simulink model "m060_HeaterAndBucket"  (R2022a)
settings: Solver=VariableStepAuto  StartTime=0.0  StopTime=500  RelTol=1e-3
settings Model: Creator=Admin  LastModifiedBy=Admin

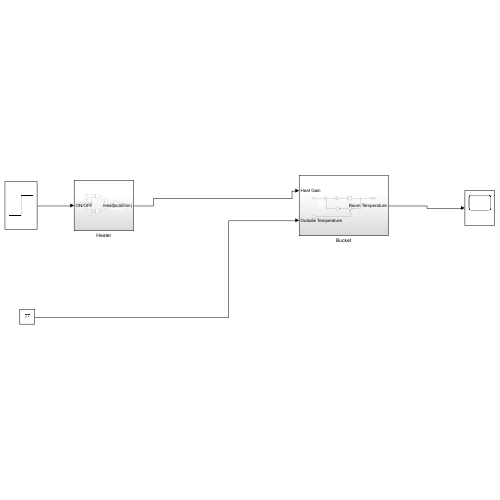
[thumbnail: Simulink's stored preview of the top-level diagram]
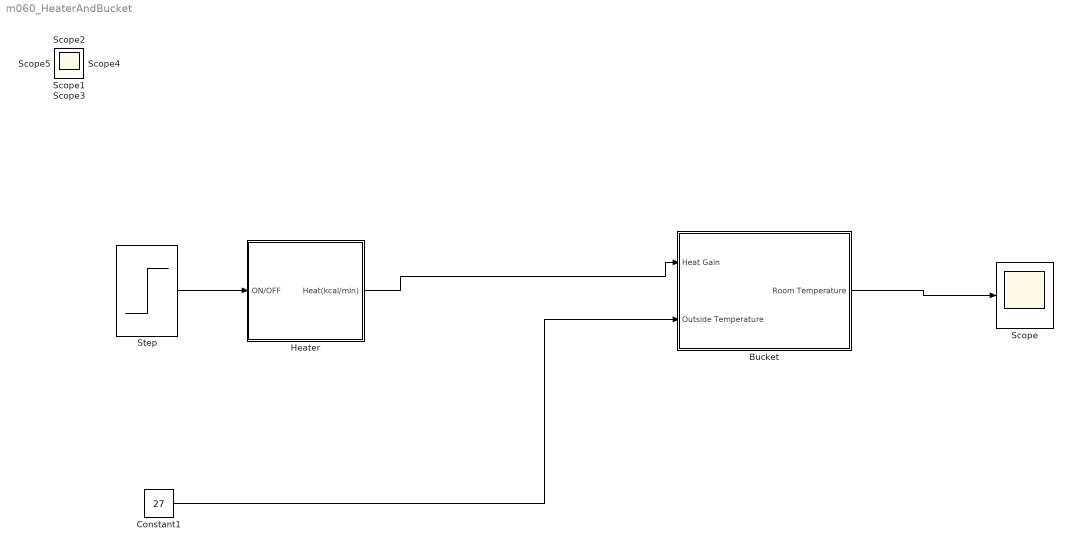
== system m060_HeaterAndBucket ==
  Bucket : Subsystem
  Constant1 : Constant  Value=27
  Heater : Subsystem
  Scope{,1..5} (6 alike) : Scope
  Step : Step  Time=3  SampleTime=0
  wires:
  Step/1 -> Heater/1(ON/OFF)
  Heater/1(Heat(kcal/min)) -> Bucket/1(Heat Gain)
  Constant1/1 -> Bucket/2(Outside Temperature)
  Bucket/1(Room Temperature) -> Scope/1

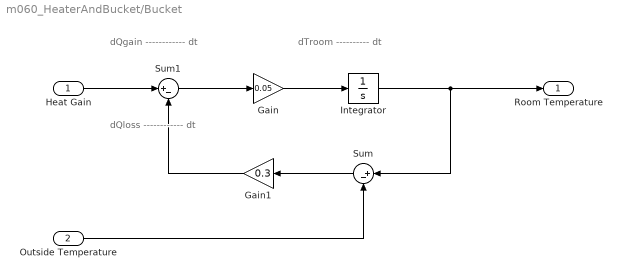
== system m060_HeaterAndBucket/Bucket ==
  note: dQgain
      | ------------
      |      dt
  note: dQloss
      | ------------
      |      dt
  note: dTroom
      | ----------
      |     dt
  Heat Gain : Inport
  Outside Temperature : Inport  Port=2
  Gain : Gain  Gain=0.05
  Gain1 : Gain  Gain=0.3
  Integrator : Integrator  InitialCondition=20
  Sum : Sum  Inputs=|+-
  Sum1 : Sum  Inputs=|+-
  Room Temperature : Outport
  wires:
  Gain/1 -> Integrator/1
  Sum/1 -> Gain1/1
  Sum1/1 -> Gain/1
  Gain1/1 -> Sum1/2
  Outside Temperature/1 -> Sum/2
  Integrator/1 -> Sum/1, Room Temperature/1
  Heat Gain/1 -> Sum1/1

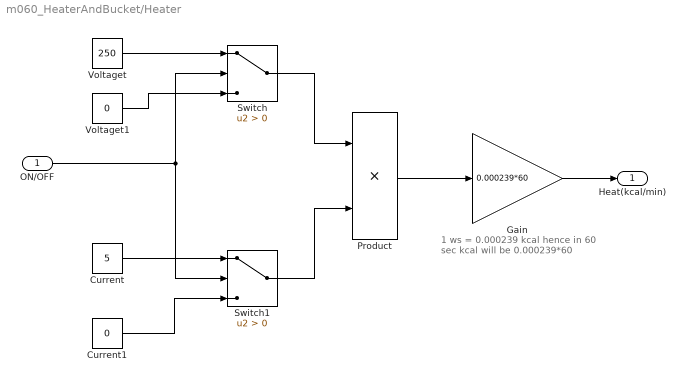
== system m060_HeaterAndBucket/Heater ==
  note: 1 ws = 0.000239 kcal hence
      | in 60 sec kcal will be 0.000239*60
  ON/OFF : Inport
  Current : Constant  Value=5
  Current1 : Constant  Value=0
  Gain : Gain  Gain=0.000239*60
  Product : Product
  Switch : Switch  Criteria=u2 > Threshold  SaturateOnIntegerOverflow=off  InputSameDT=off
  Switch1 : Switch  Criteria=u2 > Threshold  SaturateOnIntegerOverflow=off  InputSameDT=off
  Voltaget : Constant  Value=250
  Voltaget1 : Constant  Value=0
  Heat(kcal/min) : Outport
  wires:
  Gain/1 -> Heat(kcal/min)/1
  Product/1 -> Gain/1
  Voltaget/1 -> Switch/1
  Current/1 -> Switch1/1
  ON/OFF/1 -> Switch1/2, Switch/2
  Voltaget1/1 -> Switch/3
  Switch/1 -> Product/1
  Switch1/1 -> Product/2
  Current1/1 -> Switch1/3
